simulink model "Sim_Forcing_003h_expe_infra5_full_control4"  (Simulink 7.4)
settings: Solver=FixedStepDiscrete  StartTime=0.0  StopTime=inf  FixedStep=0.004  RelTol=1e-3
undefined symbols (not defined in the file or in its folder): DiscIntNeverNeededParam
libraries: simulink x28, gt_rt_lib x22, xpcutilitieslib x4, xpclib x2, dspswit3 x1
(part 2 of 4)

== system Sim_Forcing_003h_expe_infra5_full_control4/Data to Control Node 12/06/15/Interaction device from VIS (Stick)  ==
  Display2 : Display
  Display4 : Display
  Display5 : Display
  Error : Display
  GT-RT UDP  Read : gt_rt_lib/GT-RT UDP  Controller  uri='gtp://localhost/udp?port=9600'
  GT-RT UDP RX : gt_rt_lib/GT-RT UDP RX  uri='gtp://localhost/udp?port=9600'  receive_buffer_size=28  timeout=0  sample_time=0.004
  Terminator : Terminator
  Unpack : xpclib/UDP/Unpack  dimensions={3,8,1,1}  datatypes={'single','uint8','single','single'}  byteAlign=1
  Stick Out : Outport  OutDataType=fixdt(1, 16)  OutScaling=2^0
  Buttons : Outport  Port=2  OutDataType=fixdt(1, 16)  OutScaling=2^0
  Speed_Test_VIS_Send : Outport  Port=3  OutDataType=fixdt(1, 16)  OutScaling=2^0
  for_delay_calc : Outport  Port=4  OutDataType=fixdt(1, 16)  OutScaling=2^0
  wires:
  GT-RT UDP RX/2 -> Display2/1
  GT-RT UDP RX/6 -> Error/1
  GT-RT UDP RX/5 -> Display4/1
  GT-RT UDP RX/4 -> Display5/1
  GT-RT UDP RX/1 -> Unpack/1
  GT-RT UDP RX/3 -> Terminator/1
  Unpack/1 -> Stick Out/1
  Unpack/2 -> Buttons/1
  Unpack/3 -> Speed_Test_VIS_Send/1
  Unpack/4 -> for_delay_calc/1

== system Sim_Forcing_003h_expe_infra5_full_control4/Handshake CAN/If Action Subsystem ==
  Action Port : ActionPort
  GT-RT CAN TX : gt_rt_lib/GT-RT CAN TX  uri='gt_rt_dev://localhost/dev/can0#0'  mff=MFF_11_DAT
  TX CAN ID1 : Constant  Value=hex2dec('100')  OutDataTypeMode=uint32  OutDataType=sfix(16)  OutScaling=2^0  OutDataTypeStr=uint32
  TX Data : Constant  OutDataTypeMode=uint8  OutDataType=sfix(16)  OutScaling=2^0  OutDataTypeStr=uint8
  wires:
  TX CAN ID1/1 -> GT-RT CAN TX/1
  TX Data/1 -> GT-RT CAN TX/2

== system Sim_Forcing_003h_expe_infra5_full_control4/Handshake CAN/If Action Subsystem1 ==
  Action Port : ActionPort  ActionType=then
  GT-RT CAN TX : gt_rt_lib/GT-RT CAN TX  uri='gt_rt_dev://localhost/dev/can0#0'  mff=MFF_11_DAT
  TX CAN ID1 : Constant  Value=hex2dec('100')  OutDataTypeMode=uint32  OutDataType=sfix(16)  OutScaling=2^0  OutDataTypeStr=uint32
  TX Data : Constant  OutDataTypeMode=uint8  OutDataType=sfix(16)  OutScaling=2^0  OutDataTypeStr=uint8
  wires:
  TX CAN ID1/1 -> GT-RT CAN TX/1
  TX Data/1 -> GT-RT CAN TX/2

== system Sim_Forcing_003h_expe_infra5_full_control4/Joint Controller (May 7, 2015)1/Forward Kinematics ==
  J_ANG_ACT : Inport
  Data Type Conversion4 : DataTypeConversion  OutDataTypeMode=double  OutDataType=fixdt(1, 16)  OutScaling=2^0  OutDataTypeStr=double
  Demux1 : Demux  Outputs=[3,1,1,1]
  Embedded MATLAB Function : Stateflow chart
  KUKA2NED : Subsystem
  Mux : Mux  Inputs=3
  6-DOF_ACT : Outport
  roll_pitch_yaw_act : Outport  Port=2
  wires:
  KUKA2NED/1(NED) -> Embedded MATLAB Function/1(vec)
  Embedded MATLAB Function/1(out) -> 6-DOF_ACT/1, Data Type Conversion4/1
  J_ANG_ACT/1 -> KUKA2NED/1(KUKA)
  Demux1/3 -> Mux/2
  Demux1/2 -> Mux/1
  Mux/1 -> roll_pitch_yaw_act/1
  Data Type Conversion4/1 -> Demux1/1
  Demux1/4 -> Mux/3

== system Sim_Forcing_003h_expe_infra5_full_control4/Joint Controller (May 7, 2015)1/Increments ==
  J_ANG : Inport
  Sum6 : Sum  Inputs=|+-  OutDataType=fixdt(1, 16)  OutScaling=2^0
  Unit Delay6 : UnitDelay  X0=[0 50 -68 0 18 0]'  SampleTime=-1
  J_ANG_INC : Outport
  wires:
  Unit Delay6/1 -> Sum6/2
  J_ANG/1 -> Unit Delay6/1, Sum6/1
  Sum6/1 -> J_ANG_INC/1

== system Sim_Forcing_003h_expe_infra5_full_control4/Joint Controller (May 7, 2015)1/Inverse Kinematics May 6, 2015 ==
  note: Delay of 0.004s to initialize the currect step with the value of J_ANG of the previous loop
  6-DOF : Inport  OutDataType=fixdt(1, 16)  OutScaling=2^0
  Activate_full_inverse : Inport  Port=2  OutDataType=fixdt(1, 16)  OutScaling=2^0
  6_DOF_ACT : Inport  Port=3  OutDataType=fixdt(1, 16)  OutScaling=2^0
  Constant : Constant  OutDataType=fixdt(1, 16)  OutScaling=2^0
  Demux : Demux  Outputs=[6 1]
  Ground : Ground
  Inverse Kinematics : Subsystem
  Mux : Mux  Inputs=2
  NED2KUKA : Subsystem
  Scope1 : Scope
      settings: YMin=-50  YMax=70  SaveName=ScopeData4
  Simplified Inverse Kinematics : Subsystem
  Starting Joint Angles KUKA : Constant  Value=[0 -50 68 0 -18 15.89]'  OutDataType=fixdt(1, 16)  OutScaling=2^0
  Starting Joint Angles NED : Constant  Value=[0 50 -68 0 18 0]'  OutDataType=fixdt(1, 16)  OutScaling=2^0
  Switch : Switch  Criteria=u2 > Threshold  OutDataType=fixdt(1, 16)  OutScaling=2^0
  Switch1 : Switch  Criteria=u2 > Threshold  OutDataType=fixdt(1, 16)  OutScaling=2^0
  Unit Delay : UnitDelay  X0=[0 50 -68 0 18 0]'  SampleTime=-1
  J_ANG : Outport  OutDataType=fixdt(1, 16)  OutScaling=2^0
  N : Outport  Port=2  OutDataType=fixdt(1, 16)  OutScaling=2^0
  wires:
  NED2KUKA/1(KUKA) -> Scope1/1, J_ANG/1
  6-DOF/1 -> Mux/1
  Unit Delay/1 -> Mux/2
  Demux/1 -> NED2KUKA/1(NED), Unit Delay/1
  Demux/2 -> N/1
  Simplified Inverse Kinematics/1(out) -> Switch/1
  Inverse Kinematics/1(out) -> Switch/3
  Switch/1 -> Demux/1
  Mux/1 -> Inverse Kinematics/1(vec), Simplified Inverse Kinematics/2(vec)
  Activate_full_inverse/1 -> Inverse Kinematics/2(Activate full inverse), Switch1/2
  Ground/1 -> Switch1/1
  Switch1/1 -> Simplified Inverse Kinematics/1(activate simplified), Switch/2
  Constant/1 -> Switch1/3
  6_DOF_ACT/1 -> Inverse Kinematics/3(6_DOF_ACT)

== system Sim_Forcing_003h_expe_infra5_full_control4/Joint Controller (May 7, 2015)1/Subtract psi offset ==
  Psi_Offset : Inport
  J_ANG_ACT : Inport  Port=2
  Data Type Conversion : DataTypeConversion  OutDataTypeMode=double  OutDataType=fixdt(1, 16)  OutScaling=2^0  OutDataTypeStr=double
  Demux1 : Demux  Outputs=[1,5]
  Mux1 : Mux  Inputs=[1,5]
  Sum3 : Sum  Inputs=-+|  OutDataType=fixdt(1, 16)  OutScaling=2^0
  out : Outport
  wires:
  Demux1/1 -> Sum3/2
  Sum3/1 -> Mux1/1
  Demux1/2 -> Mux1/2
  J_ANG_ACT/1 -> Data Type Conversion/1
  Mux1/1 -> out/1
  Data Type Conversion/1 -> Demux1/1
  Psi_Offset/1 -> Sum3/1

== system Sim_Forcing_003h_expe_infra5_full_control4/BEC (May 7, 2015)/CAN Receive/Convert 4*uni8 to int ==
  byte0 : Inport
  byte1 : Inport  Port=2
  byte2 : Inport  Port=3
  byte3 : Inport  Port=4
  Add : Sum  Inputs=++++  OutDataTypeMode=int32  OutDataType=fixdt(1, 16)  OutScaling=2^-10  OutDataTypeStr=int32
  Gain2 : Gain  Gain=256  ParameterDataType=fixdt(1, 16)  ParameterScaling=2^0  OutDataType=fixdt(1, 16)  OutScaling=2^0
  Gain3 : Gain  Gain=2^16  ParameterDataType=fixdt(1, 16)  ParameterScaling=2^0  OutDataType=fixdt(1, 16)  OutScaling=2^0
  Gain4 : Gain  Gain=2^24  ParameterDataType=fixdt(1, 16)  ParameterScaling=2^0  OutDataType=fixdt(1, 16)  OutScaling=2^0
  int : Outport
  wires:
  Gain2/1 -> Add/2
  Gain3/1 -> Add/3
  byte0/1 -> Add/1
  Add/1 -> int/1
  byte1/1 -> Gain2/1
  byte2/1 -> Gain3/1
  byte3/1 -> Gain4/1
  Gain4/1 -> Add/4

== system Sim_Forcing_003h_expe_infra5_full_control4/BEC (May 7, 2015)/CAN Receive/Convert 4*uni8 to int1 ==
  byte0 : Inport
  byte1 : Inport  Port=2
  byte2 : Inport  Port=3
  byte3 : Inport  Port=4
  Add : Sum  Inputs=++++  OutDataTypeMode=int32  OutDataType=fixdt(1, 16)  OutScaling=2^-10  OutDataTypeStr=int32
  Gain2 : Gain  Gain=256  ParameterDataType=fixdt(1, 16)  ParameterScaling=2^0  OutDataType=fixdt(1, 16)  OutScaling=2^0
  Gain3 : Gain  Gain=2^16  ParameterDataType=fixdt(1, 16)  ParameterScaling=2^0  OutDataType=fixdt(1, 16)  OutScaling=2^0
  Gain4 : Gain  Gain=2^24  ParameterDataType=fixdt(1, 16)  ParameterScaling=2^0  OutDataType=fixdt(1, 16)  OutScaling=2^0
  int : Outport
  wires:
  Gain4/1 -> Add/4
  byte3/1 -> Gain4/1
  byte2/1 -> Gain3/1
  byte1/1 -> Gain2/1
  Add/1 -> int/1
  byte0/1 -> Add/1
  Gain3/1 -> Add/3
  Gain2/1 -> Add/2

== system Sim_Forcing_003h_expe_infra5_full_control4/BEC (May 7, 2015)/CAN Receive/Convert 4*uni8 to int2 ==
  byte0 : Inport
  byte1 : Inport  Port=2
  byte2 : Inport  Port=3
  byte3 : Inport  Port=4
  Add : Sum  Inputs=++++  OutDataTypeMode=int32  OutDataType=fixdt(1, 16)  OutScaling=2^-10  OutDataTypeStr=int32
  Gain2 : Gain  Gain=256  ParameterDataType=fixdt(1, 16)  ParameterScaling=2^0  OutDataType=fixdt(1, 16)  OutScaling=2^0
  Gain3 : Gain  Gain=2^16  ParameterDataType=fixdt(1, 16)  ParameterScaling=2^0  OutDataType=fixdt(1, 16)  OutScaling=2^0
  Gain4 : Gain  Gain=2^24  ParameterDataType=fixdt(1, 16)  ParameterScaling=2^0  OutDataType=fixdt(1, 16)  OutScaling=2^0
  int : Outport
  wires:
  Gain2/1 -> Add/2
  Gain3/1 -> Add/3
  byte0/1 -> Add/1
  Add/1 -> int/1
  byte1/1 -> Gain2/1
  byte2/1 -> Gain3/1
  byte3/1 -> Gain4/1
  Gain4/1 -> Add/4

== system Sim_Forcing_003h_expe_infra5_full_control4/BEC (May 7, 2015)/CAN Receive/Convert 4*uni8 to int3 ==
  byte0 : Inport
  byte1 : Inport  Port=2
  byte2 : Inport  Port=3
  byte3 : Inport  Port=4
  Add : Sum  Inputs=++++  OutDataTypeMode=int32  OutDataType=fixdt(1, 16)  OutScaling=2^-10  OutDataTypeStr=int32
  Gain2 : Gain  Gain=256  ParameterDataType=fixdt(1, 16)  ParameterScaling=2^0  OutDataType=fixdt(1, 16)  OutScaling=2^0
  Gain3 : Gain  Gain=2^16  ParameterDataType=fixdt(1, 16)  ParameterScaling=2^0  OutDataType=fixdt(1, 16)  OutScaling=2^0
  Gain4 : Gain  Gain=2^24  ParameterDataType=fixdt(1, 16)  ParameterScaling=2^0  OutDataType=fixdt(1, 16)  OutScaling=2^0
  int : Outport
  wires:
  Gain4/1 -> Add/4
  byte3/1 -> Gain4/1
  byte2/1 -> Gain3/1
  byte1/1 -> Gain2/1
  Add/1 -> int/1
  byte0/1 -> Add/1
  Gain3/1 -> Add/3
  Gain2/1 -> Add/2

== system Sim_Forcing_003h_expe_infra5_full_control4/BEC (May 7, 2015)/CAN Receive/Convert 4*uni8 to int4 ==
  byte0 : Inport
  byte1 : Inport  Port=2
  byte2 : Inport  Port=3
  byte3 : Inport  Port=4
  Add : Sum  Inputs=++++  OutDataTypeMode=int32  OutDataType=fixdt(1, 16)  OutScaling=2^-10  OutDataTypeStr=int32
  Gain2 : Gain  Gain=256  ParameterDataType=fixdt(1, 16)  ParameterScaling=2^0  OutDataType=fixdt(1, 16)  OutScaling=2^0
  Gain3 : Gain  Gain=2^16  ParameterDataType=fixdt(1, 16)  ParameterScaling=2^0  OutDataType=fixdt(1, 16)  OutScaling=2^0
  Gain4 : Gain  Gain=2^24  ParameterDataType=fixdt(1, 16)  ParameterScaling=2^0  OutDataType=fixdt(1, 16)  OutScaling=2^0
  int : Outport
  wires:
  Gain2/1 -> Add/2
  Gain3/1 -> Add/3
  byte0/1 -> Add/1
  Add/1 -> int/1
  byte1/1 -> Gain2/1
  byte2/1 -> Gain3/1
  byte3/1 -> Gain4/1
  Gain4/1 -> Add/4

== system Sim_Forcing_003h_expe_infra5_full_control4/BEC (May 7, 2015)/CAN Receive/Convert 4*uni8 to int5 ==
  byte0 : Inport
  byte1 : Inport  Port=2
  byte2 : Inport  Port=3
  byte3 : Inport  Port=4
  Add : Sum  Inputs=++++  OutDataTypeMode=int32  OutDataType=fixdt(1, 16)  OutScaling=2^-10  OutDataTypeStr=int32
  Gain2 : Gain  Gain=256  ParameterDataType=fixdt(1, 16)  ParameterScaling=2^0  OutDataType=fixdt(1, 16)  OutScaling=2^0
  Gain3 : Gain  Gain=2^16  ParameterDataType=fixdt(1, 16)  ParameterScaling=2^0  OutDataType=fixdt(1, 16)  OutScaling=2^0
  Gain4 : Gain  Gain=2^24  ParameterDataType=fixdt(1, 16)  ParameterScaling=2^0  OutDataType=fixdt(1, 16)  OutScaling=2^0
  int : Outport
  wires:
  Gain4/1 -> Add/4
  byte3/1 -> Gain4/1
  byte2/1 -> Gain3/1
  byte1/1 -> Gain2/1
  Add/1 -> int/1
  byte0/1 -> Add/1
  Gain3/1 -> Add/3
  Gain2/1 -> Add/2

== system Sim_Forcing_003h_expe_infra5_full_control4/BEC (May 7, 2015)/CAN Send/If Action Subsystem1 ==
  In1 : Inport  OutDataType=fixdt(1, 16)  OutScaling=2^0
  In2 : Inport  Port=2  OutDataType=fixdt(1, 16)  OutScaling=2^0
  In3 : Inport  Port=3  OutDataType=fixdt(1, 16)  OutScaling=2^0
  In4 : Inport  Port=4  OutDataType=fixdt(1, 16)  OutScaling=2^0
  In5 : Inport  Port=5  OutDataType=fixdt(1, 16)  OutScaling=2^0
  In6 : Inport  Port=6  OutDataType=fixdt(1, 16)  OutScaling=2^0
  Action Port : ActionPort  ActionType=then
  "Convert int to 4*uni8 " : Subsystem
  Convert int to 4*uni8 1 : Subsystem
  Convert int to 4*uni8 2 : Subsystem
  Convert int to 4*uni8 3 : Subsystem
  Convert int to 4*uni8 4 : Subsystem
  Convert int to 4*uni8 5 : Subsystem
  GT-RT CAN TX : gt_rt_lib/GT-RT CAN TX  uri='gt_rt_dev://localhost/dev/can0#0'  mff=MFF_11_DAT
  GT-RT CAN TX1 : gt_rt_lib/GT-RT CAN TX  uri='gt_rt_dev://localhost/dev/can0#0'  mff=MFF_11_DAT
  GT-RT CAN TX2 : gt_rt_lib/GT-RT CAN TX  uri='gt_rt_dev://localhost/dev/can0#0'  mff=MFF_11_DAT
  Mux : Mux  Inputs=2
  Mux1 : Mux  Inputs=2
  Mux2 : Mux  Inputs=2
  TX CAN ID1 : Constant  Value=hex2dec('101')  OutDataTypeMode=uint32  OutDataType=sfix(16)  OutScaling=2^0  OutDataTypeStr=uint32
  TX CAN ID2 : Constant  Value=hex2dec('102')  OutDataTypeMode=uint32  OutDataType=sfix(16)  OutScaling=2^0  OutDataTypeStr=uint32
  TX CAN ID3 : Constant  Value=hex2dec('103')  OutDataTypeMode=uint32  OutDataType=sfix(16)  OutScaling=2^0  OutDataTypeStr=uint32
  wires:
  In1/1 -> "Convert int to 4*uni8 "/1(in)
  In2/1 -> Convert int to 4*uni8 1/1(in)
  In3/1 -> Convert int to 4*uni8 2/1(in)
  In4/1 -> Convert int to 4*uni8 3/1(in)
  In5/1 -> Convert int to 4*uni8 4/1(in)
  In6/1 -> Convert int to 4*uni8 5/1(in)
  Mux2/1 -> GT-RT CAN TX2/2
  Convert int to 4*uni8 5/1(out) -> Mux2/2
  Convert int to 4*uni8 4/1(out) -> Mux2/1
  Mux1/1 -> GT-RT CAN TX1/2
  Convert int to 4*uni8 3/1(out) -> Mux1/2
  Convert int to 4*uni8 2/1(out) -> Mux1/1
  Mux/1 -> GT-RT CAN TX/2
  Convert int to 4*uni8 1/1(out) -> Mux/2
  "Convert int to 4*uni8 "/1(out) -> Mux/1
  TX CAN ID3/1 -> GT-RT CAN TX2/1
  TX CAN ID2/1 -> GT-RT CAN TX1/1
  TX CAN ID1/1 -> GT-RT CAN TX/1

== system Sim_Forcing_003h_expe_infra5_full_control4/BEC (May 7, 2015)/Software limit switches/Subsystem ==
  In1 : Inport
  act : Inport  Port=2
  Abs1 : Abs  OutDataType=fixdt(1, 16)  OutScaling=2^0
  Abs2 : Abs  OutDataType=fixdt(1, 16)  OutScaling=2^0
  Add1 : Sum  Inputs=+-  OutDataType=fixdt(1, 16)  OutScaling=2^-10
  Add2 : Sum  Inputs=-+  OutDataType=fixdt(1, 16)  OutScaling=2^-10
  Display : Display
  Display2 : Display
  If Action Subsystem : Subsystem  TreatAsAtomicUnit=on
  If Action Subsystem1 : Subsystem  TreatAsAtomicUnit=on
  If2 : If
  NSEA1 : Constant  Value=-160  OutDataType=fixdt(1, 16)  OutScaling=2^0
  PSEA1 : Constant  Value=160  OutDataType=fixdt(1, 16)  OutScaling=2^0
  Switch : Switch  Criteria=u2 > Threshold  OutDataType=fixdt(1, 16)  OutScaling=2^0
  Switch1 : Switch  Criteria=u2 ~= 0  OutDataType=fixdt(1, 16)  OutScaling=2^0
  Out1 : Outport
  wires:
  If Action Subsystem1/1(Out1) -> Switch/3
  If Action Subsystem/1(Out1) -> Display/1, Switch/1
  Abs1/1 -> If Action Subsystem1/2(dif)
  If2/2 -> If Action Subsystem1/Action
  If2/1 -> If Action Subsystem/Action
  In1/1 -> If2/1, If Action Subsystem/2(Inc), If Action Subsystem1/1(Inc), Switch/2, Switch1/2, Switch1/3
  Abs2/1 -> If Action Subsystem/1(dif)
  NSEA1/1 -> Add1/2
  PSEA1/1 -> Add2/1
  Add1/1 -> Abs1/1
  Add2/1 -> Abs2/1
  Switch/1 -> Switch1/1
  Switch1/1 -> Out1/1, Display2/1
  act/1 -> Add1/1, Add2/2

== system Sim_Forcing_003h_expe_infra5_full_control4/BEC (May 7, 2015)/Software limit switches/Subsystem1 ==
  In1 : Inport
  act : Inport  Port=2
  Abs1 : Abs  OutDataType=fixdt(1, 16)  OutScaling=2^0
  Abs2 : Abs  OutDataType=fixdt(1, 16)  OutScaling=2^0
  Add1 : Sum  Inputs=+-  OutDataType=fixdt(1, 16)  OutScaling=2^-10
  Add2 : Sum  Inputs=-+  OutDataType=fixdt(1, 16)  OutScaling=2^-10
  If Action Subsystem : Subsystem  TreatAsAtomicUnit=on
  If Action Subsystem1 : Subsystem  TreatAsAtomicUnit=on
  If2 : If
  NSEA1 : Constant  Value=-130  OutDataType=fixdt(1, 16)  OutScaling=2^0
  PSEA1 : Constant  Value=20  OutDataType=fixdt(1, 16)  OutScaling=2^0
  Switch : Switch  OutDataType=fixdt(1, 16)  OutScaling=2^0
  Switch1 : Switch  Criteria=u2 ~= 0  OutDataType=fixdt(1, 16)  OutScaling=2^0
  Out1 : Outport
  wires:
  act/1 -> Add1/1, Add2/2
  Add2/1 -> Abs2/1
  Add1/1 -> Abs1/1
  PSEA1/1 -> Add2/1
  NSEA1/1 -> Add1/2
  Abs2/1 -> If Action Subsystem/1(dif)
  In1/1 -> If Action Subsystem1/1(Inc), If Action Subsystem/2(Inc), Switch/2, Switch1/2, Switch1/3, If2/1
  If2/1 -> If Action Subsystem/Action
  If2/2 -> If Action Subsystem1/Action
  Abs1/1 -> If Action Subsystem1/2(dif)
  If Action Subsystem/1(Out1) -> Switch/1
  If Action Subsystem1/1(Out1) -> Switch/3
  Switch/1 -> Switch1/1
  Switch1/1 -> Out1/1

== system Sim_Forcing_003h_expe_infra5_full_control4/BEC (May 7, 2015)/Software limit switches/Subsystem2 ==
  In1 : Inport
  act : Inport  Port=2
  Abs1 : Abs  OutDataType=fixdt(1, 16)  OutScaling=2^0
  Abs2 : Abs  OutDataType=fixdt(1, 16)  OutScaling=2^0
  Add1 : Sum  Inputs=+-  OutDataType=fixdt(1, 16)  OutScaling=2^-10
  Add2 : Sum  Inputs=-+  OutDataType=fixdt(1, 16)  OutScaling=2^-10
  If Action Subsystem : Subsystem  TreatAsAtomicUnit=on
  If Action Subsystem1 : Subsystem  TreatAsAtomicUnit=on
  If2 : If
  NSEA1 : Constant  Value=-88  OutDataType=fixdt(1, 16)  OutScaling=2^0
  PSEA1 : Constant  Value=88  OutDataType=fixdt(1, 16)  OutScaling=2^0
  Switch : Switch  OutDataType=fixdt(1, 16)  OutScaling=2^0
  Switch1 : Switch  Criteria=u2 ~= 0  OutDataType=fixdt(1, 16)  OutScaling=2^0
  Out1 : Outport
  wires:
  If Action Subsystem1/1(Out1) -> Switch/3
  If Action Subsystem/1(Out1) -> Switch/1
  Abs1/1 -> If Action Subsystem1/2(dif)
  If2/2 -> If Action Subsystem1/Action
  If2/1 -> If Action Subsystem/Action
  In1/1 -> If2/1, If Action Subsystem/2(Inc), If Action Subsystem1/1(Inc), Switch/2, Switch1/2, Switch1/3
  Abs2/1 -> If Action Subsystem/1(dif)
  NSEA1/1 -> Add1/2
  PSEA1/1 -> Add2/1
  Add1/1 -> Abs1/1
  Add2/1 -> Abs2/1
  act/1 -> Add1/1, Add2/2
  Switch/1 -> Switch1/1
  Switch1/1 -> Out1/1

== system Sim_Forcing_003h_expe_infra5_full_control4/BEC (May 7, 2015)/Software limit switches/Subsystem3 ==
  In1 : Inport
  act : Inport  Port=2
  Abs1 : Abs  OutDataType=fixdt(1, 16)  OutScaling=2^0
  Abs2 : Abs  OutDataType=fixdt(1, 16)  OutScaling=2^0
  Add1 : Sum  Inputs=+-  OutDataType=fixdt(1, 16)  OutScaling=2^-10
  Add2 : Sum  Inputs=-+  OutDataType=fixdt(1, 16)  OutScaling=2^-10
  If Action Subsystem : Subsystem  TreatAsAtomicUnit=on
  If Action Subsystem1 : Subsystem  TreatAsAtomicUnit=on
  If2 : If
  NSEA1 : Constant  Value=-350  OutDataType=fixdt(1, 16)  OutScaling=2^0
  PSEA1 : Constant  Value=350  OutDataType=fixdt(1, 16)  OutScaling=2^0
  Switch : Switch  OutDataType=fixdt(1, 16)  OutScaling=2^0
  Switch1 : Switch  Criteria=u2 ~= 0  OutDataType=fixdt(1, 16)  OutScaling=2^0
  Out1 : Outport
  wires:
  Add2/1 -> Abs2/1
  Add1/1 -> Abs1/1
  PSEA1/1 -> Add2/1
  NSEA1/1 -> Add1/2
  Abs2/1 -> If Action Subsystem/1(dif)
  In1/1 -> If Action Subsystem1/1(Inc), If Action Subsystem/2(Inc), Switch/2, Switch1/2, Switch1/3, If2/1
  If2/1 -> If Action Subsystem/Action
  If2/2 -> If Action Subsystem1/Action
  act/1 -> Add2/2, Add1/1
  Abs1/1 -> If Action Subsystem1/2(dif)
  If Action Subsystem/1(Out1) -> Switch/1
  If Action Subsystem1/1(Out1) -> Switch/3
  Switch/1 -> Switch1/1
  Switch1/1 -> Out1/1

== system Sim_Forcing_003h_expe_infra5_full_control4/BEC (May 7, 2015)/Software limit switches/Subsystem4 ==
  In1 : Inport
  act : Inport  Port=2
  Abs1 : Abs  OutDataType=fixdt(1, 16)  OutScaling=2^0
  Abs2 : Abs  OutDataType=fixdt(1, 16)  OutScaling=2^0
  Add1 : Sum  Inputs=+-  OutDataType=fixdt(1, 16)  OutScaling=2^-10
  Add2 : Sum  Inputs=-+  OutDataType=fixdt(1, 16)  OutScaling=2^-10
  If Action Subsystem : Subsystem  TreatAsAtomicUnit=on
  If Action Subsystem1 : Subsystem  TreatAsAtomicUnit=on
  If2 : If
  NSEA1 : Constant  Value=-61  OutDataType=fixdt(1, 16)  OutScaling=2^0
  PSEA1 : Constant  Value=61  OutDataType=fixdt(1, 16)  OutScaling=2^0
  Switch : Switch  OutDataType=fixdt(1, 16)  OutScaling=2^0
  Switch1 : Switch  Criteria=u2 ~= 0  OutDataType=fixdt(1, 16)  OutScaling=2^0
  Out1 : Outport
  wires:
  If Action Subsystem/1(Out1) -> Switch/1
  Abs1/1 -> If Action Subsystem1/2(dif)
  If2/2 -> If Action Subsystem1/Action
  If2/1 -> If Action Subsystem/Action
  In1/1 -> If2/1, If Action Subsystem/2(Inc), If Action Subsystem1/1(Inc), Switch/2, Switch1/2, Switch1/3
  Abs2/1 -> If Action Subsystem/1(dif)
  NSEA1/1 -> Add1/2
  PSEA1/1 -> Add2/1
  Add1/1 -> Abs1/1
  Add2/1 -> Abs2/1
  If Action Subsystem1/1(Out1) -> Switch/3
  Switch/1 -> Switch1/1
  Switch1/1 -> Out1/1
  act/1 -> Add2/2, Add1/1

== system Sim_Forcing_003h_expe_infra5_full_control4/BEC (May 7, 2015)/Software limit switches/Subsystem5 ==
  In1 : Inport
  act : Inport  Port=2
  Abs1 : Abs  OutDataType=fixdt(1, 16)  OutScaling=2^0
  Abs2 : Abs  OutDataType=fixdt(1, 16)  OutScaling=2^0
  Add1 : Sum  Inputs=+-  OutDataType=fixdt(1, 16)  OutScaling=2^-10
  Add2 : Sum  Inputs=-+  OutDataType=fixdt(1, 16)  OutScaling=2^-10
  If Action Subsystem : Subsystem  TreatAsAtomicUnit=on
  If Action Subsystem1 : Subsystem  TreatAsAtomicUnit=on
  If2 : If
  NSEA1 : Constant  Value=-350  OutDataType=fixdt(1, 16)  OutScaling=2^0
  PSEA1 : Constant  Value=350  OutDataType=fixdt(1, 16)  OutScaling=2^0
  Switch : Switch  OutDataType=fixdt(1, 16)  OutScaling=2^0
  Switch1 : Switch  Criteria=u2 ~= 0  OutDataType=fixdt(1, 16)  OutScaling=2^0
  Out1 : Outport
  wires:
  Add2/1 -> Abs2/1
  Add1/1 -> Abs1/1
  PSEA1/1 -> Add2/1
  NSEA1/1 -> Add1/2
  Abs2/1 -> If Action Subsystem/1(dif)
  In1/1 -> If Action Subsystem1/1(Inc), If Action Subsystem/2(Inc), Switch/2, Switch1/2, Switch1/3, If2/1
  If2/1 -> If Action Subsystem/Action
  If2/2 -> If Action Subsystem1/Action
  Abs1/1 -> If Action Subsystem1/2(dif)
  If Action Subsystem/1(Out1) -> Switch/1
  If Action Subsystem1/1(Out1) -> Switch/3
  Switch/1 -> Switch1/1
  Switch1/1 -> Out1/1
  act/1 -> Add2/2, Add1/1

== system Sim_Forcing_003h_expe_infra5_full_control4/Breaking_Control 20/07/15/Move UP1/Smooth Displacement Second-Order Filter, zeta 0.8 ==
  Step IN Reset on  either : Inport
  T : Inport  Port=2  OutDataType=fixdt(1, 16)  OutScaling=2^0
  (zeta*T_transfer)/pi : Gain  Gain=0.8/pi  ParameterDataType=fixdt(1, 16)  ParameterScaling=2^0  OutDataType=fixdt(1, 16)  OutScaling=2^0
  4*zeta*pi : Gain  Gain=3.2*pi  ParameterDataType=fixdt(1, 16)  ParameterScaling=2^0  OutDataType=fixdt(1, 16)  OutScaling=2^0
  4*zeta*pi/T_transfer /s : DiscreteIntegrator  gainval=1  ExternalReset=either  InitialConditionSource=external  SampleTime=0.004  OutDataType=fixdt(1, 16)  OutScaling=2^0  ICPrevOutput=DiscIntNeverNeededParam  ICPrevScaledInput=DiscIntNeverNeededParam
  Discrete Derivative : simulink/Discrete/Discrete Derivative  SystemSampleTime=-1  gainval=1.0  ICPrevScaledInput=0.0  OutMin=[]  OutMax=[]  OutDataType=fixdt(1, 16)  OutScaling=2^-10  DoSatur=off
  Divide : Product  Inputs=*/  OutDataType=fixdt(1, 16)  OutScaling=2^-10
  Divide1 : Product  Inputs=*/  OutDataType=fixdt(1, 16)  OutScaling=2^-10
  For saving position  and velocity until after switchover : UnitDelay  SampleTime=-1
  Product : Product  OutDataType=fixdt(1, 16)  OutScaling=2^0  RndMeth=Zero
  Sum1 : Sum  Inputs=|+-  OutDataType=fixdt(1, 16)  OutScaling=2^0
  Sum2 : Sum  Inputs=-+|  OutDataType=fixdt(1, 16)  OutScaling=2^0
  pi/(zeta*T_transfer)/s : DiscreteIntegrator  gainval=1  ExternalReset=either  InitialConditionSource=external  SampleTime=0.004  OutDataType=fixdt(1, 16)  OutScaling=2^0  ICPrevOutput=DiscIntNeverNeededParam  ICPrevScaledInput=DiscIntNeverNeededParam
  pi/zeta : Gain  Gain=pi/0.8  ParameterDataType=fixdt(1, 16)  ParameterScaling=2^0  OutDataType=fixdt(1, 16)  OutScaling=2^0
  Out : Outport
  wires:
  Discrete Derivative/1 -> Product/2
  Product/1 -> (zeta*T_transfer)/pi/1
  Divide/1 -> 4*zeta*pi/1
  Divide1/1 -> pi/zeta/1
  pi/zeta/1 -> pi/(zeta*T_transfer)/s/1
  pi/(zeta*T_transfer)/s/1 -> Sum2/1, Out/1, For saving position  and velocity until after switchover/1
  4*zeta*pi/T_transfer /s/1 -> Divide1/1, Sum1/2
  Sum1/1 -> Divide/1
  4*zeta*pi/1 -> 4*zeta*pi/T_transfer /s/1
  T/1 -> [T]
  Step IN Reset on  either/1 -> [Step], Sum2/2
  [Step] -> 4*zeta*pi/T_transfer /s/2
  [Step] -> pi/(zeta*T_transfer)/s/2
  [T] -> Divide/2
  For saving position  and velocity until after switchover/1 -> Discrete Derivative/1, pi/(zeta*T_transfer)/s/3
  [T] -> Product/1
  (zeta*T_transfer)/pi/1 -> 4*zeta*pi/T_transfer /s/3
  [T] -> Divide1/2
  Sum2/1 -> Sum1/1

== system Sim_Forcing_003h_expe_infra5_full_control4/Breaking_Control 20/07/15/Move UP1/add x_offset ==
  x_offset : Inport
  set_in : Inport  Port=2
  Embedded MATLAB Function : Stateflow chart
  set_out : Outport
  wires:
  x_offset/1 -> Embedded MATLAB Function/1(dx)
  Embedded MATLAB Function/1(set_out) -> set_out/1
  set_in/1 -> Embedded MATLAB Function/2(set_in)

== system Sim_Forcing_003h_expe_infra5_full_control4/Breaking_Control 20/07/15/Move_cabin/Subsystem ==
  com_or : Inport
  start_zeroing : Inport  Port=2
  connect_x : Inport  Port=3
  connect_z : Inport  Port=4
  Display4 : Display
  Display5 : Display
  Embedded MATLAB Function3 : Stateflow chart
  Fcn : Fcn  Expr=abs(u(1))+abs(u(2))+abs(u(3))+abs(u(4))
  Logical Operator : Logic  AllPortsSameDT=off  OutDataTypeMode=boolean  LogicDataType=fixdt(0, 8)  OutDataTypeStr=boolean
  Logical Operator1 : Logic  Operator=OR  AllPortsSameDT=off  OutDataTypeMode=boolean  LogicDataType=fixdt(0, 8)  OutDataTypeStr=boolean
  Logical Operator2 : Logic  Operator=NOT  AllPortsSameDT=off  OutDataTypeMode=boolean  LogicDataType=fixdt(0, 8)  OutDataTypeStr=boolean
  Logical Operator3 : Logic  AllPortsSameDT=off  OutDataTypeMode=boolean  LogicDataType=fixdt(0, 8)  OutDataTypeStr=boolean
  Logical Operator4 : Logic  AllPortsSameDT=off  OutDataTypeMode=boolean  LogicDataType=fixdt(0, 8)  OutDataTypeStr=boolean
  Logical Operator5 : Logic  Operator=OR  AllPortsSameDT=off  OutDataTypeMode=boolean  LogicDataType=fixdt(0, 8)  OutDataTypeStr=boolean
  Logical Operator6 : Logic  Operator=NOT  AllPortsSameDT=off  OutDataTypeMode=boolean  LogicDataType=fixdt(0, 8)  OutDataTypeStr=boolean
  Relational Operator : RelationalOperator  Operator=<=  LogicOutDataTypeMode=boolean  LogicDataType=fixdt(0, 8)  OutDataTypeStr=boolean
  gain : Constant  Value=0.004
  flag_reset : Outport  OutDataType=fixdt(1, 16)  OutScaling=2^0
  wires:
  gain/1 -> Relational Operator/2
  Logical Operator/1 -> Display4/1, flag_reset/1
  com_or/1 -> Embedded MATLAB Function3/1(com_or), Fcn/1
  Embedded MATLAB Function3/1(max_tilt) -> Relational Operator/1
  start_zeroing/1 -> Logical Operator3/1, Logical Operator5/1
  connect_x/1 -> Logical Operator6/1, Logical Operator3/2
  connect_z/1 -> Logical Operator2/1
  Logical Operator2/1 -> Logical Operator1/2
  Logical Operator3/1 -> Logical Operator1/1
  Logical Operator1/1 -> Logical Operator/2
  Relational Operator/1 -> Logical Operator4/1
  Logical Operator4/1 -> Logical Operator/1
  Logical Operator5/1 -> Logical Operator4/2
  Logical Operator6/1 -> Logical Operator5/2

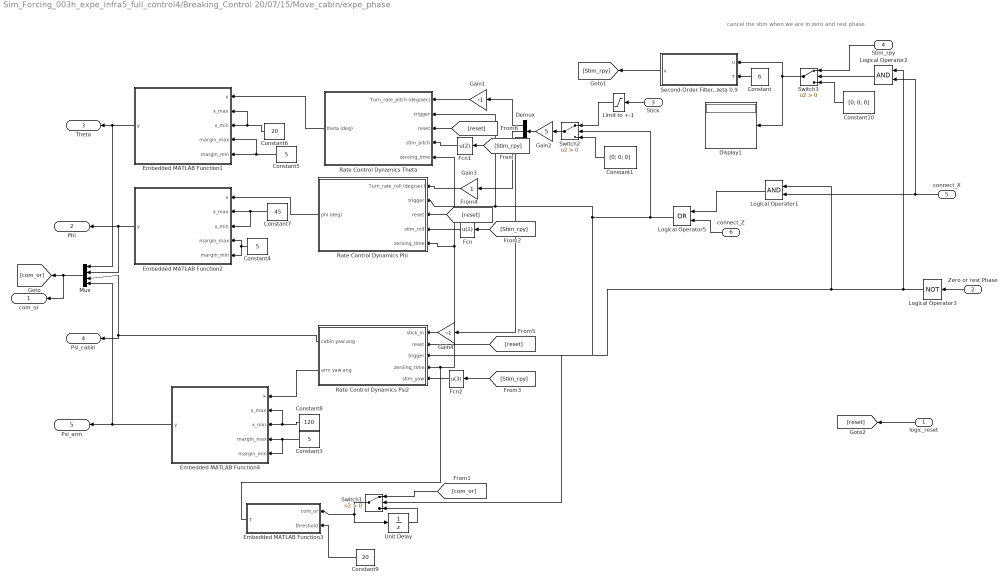
== system Sim_Forcing_003h_expe_infra5_full_control4/Breaking_Control 20/07/15/Move_cabin/expe_phase ==
  note: cancel the stim when we are in zero and rest phase
  logic_reset : Inport
  Zero or rest Phase : Inport  Port=2  OutDataType=fixdt(1, 16)  OutScaling=2^0
  Stick : Inport  Port=3
  Stim_rpy : Inport  Port=4
  connect_X : Inport  Port=5  OutDataType=fixdt(1, 16)  OutScaling=2^0
  connect_Z : Inport  Port=6  OutDataType=fixdt(1, 16)  OutScaling=2^0
  Constant : Constant  Value=6  OutDataType=fixdt(1, 16)  OutScaling=2^0
  Constant1 : Constant  Value=[0; 0; 0]  OutDataType=fixdt(1, 16)  OutScaling=2^0
  Constant10 : Constant  Value=[0; 0; 0]  OutDataType=fixdt(1, 16)  OutScaling=2^0
  Constant3 : Constant  Value=5  OutDataType=fixdt(1, 16)  OutScaling=2^0
  Constant4 : Constant  Value=5  OutDataType=fixdt(1, 16)  OutScaling=2^0
  Constant5 : Constant  Value=5  OutDataType=fixdt(1, 16)  OutScaling=2^0
  Constant6 : Constant  Value=20  OutDataType=fixdt(1, 16)  OutScaling=2^0
  Constant7 : Constant  Value=45  OutDataType=fixdt(1, 16)  OutScaling=2^0
  Constant8 : Constant  Value=120  OutDataType=fixdt(1, 16)  OutScaling=2^0
  Constant9 : Constant  Value=20  OutDataType=fixdt(1, 16)  OutScaling=2^0
  Demux : Demux  Outputs=3
  Display1 : Display
  Embedded MATLAB Function1 : Stateflow chart
  Embedded MATLAB Function2 : Stateflow chart
  Embedded MATLAB Function3 : Stateflow chart
  Embedded MATLAB Function4 : Stateflow chart
  Fcn : Fcn  Expr=u(1)
  Fcn1 : Fcn  Expr=u(2)
  Fcn2 : Fcn  Expr=u(3)
  Gain1 : Gain  Gain=-1  ParameterDataType=fixdt(1, 16)  ParameterScaling=2^0  OutDataType=fixdt(1, 16)  OutScaling=2^0
  Gain2 : Gain  Gain=5  ParameterDataType=fixdt(1, 16)  ParameterScaling=2^0  OutDataType=fixdt(1, 16)  OutScaling=2^0
  Gain3 : Gain  ParameterDataType=fixdt(1, 16)  ParameterScaling=2^0  OutDataType=fixdt(1, 16)  OutScaling=2^0
  Gain4 : Gain  Gain=-1  ParameterDataType=fixdt(1, 16)  ParameterScaling=2^0  OutDataType=fixdt(1, 16)  OutScaling=2^0
  Limit to +-1 : Saturate  UpperLimit=1  LowerLimit=-1  OutDataType=fixdt(1, 16)  OutScaling=2^0
  Logical Operator1 : Logic  AllPortsSameDT=off  OutDataTypeMode=boolean  LogicDataType=fixdt(0, 8)  OutDataTypeStr=boolean
  Logical Operator2 : Logic  AllPortsSameDT=off  OutDataTypeMode=boolean  LogicDataType=fixdt(0, 8)  OutDataTypeStr=boolean
  Logical Operator3 : Logic  Operator=NOT  AllPortsSameDT=off  OutDataTypeMode=boolean  LogicDataType=fixdt(0, 8)  OutDataTypeStr=boolean
  Logical Operator5 : Logic  Operator=OR  AllPortsSameDT=off  OutDataTypeMode=boolean  LogicDataType=fixdt(0, 8)  OutDataTypeStr=boolean
  Mux : Mux
  Rate Control Dynamics Phi : Subsystem
  Rate Control Dynamics Psi2 : Subsystem
  Rate Control Dynamics Theta : Subsystem
  "Second-Order Filter, zeta 0.9" : Subsystem
  Switch1 : Switch  Criteria=u2 > Threshold  OutDataType=fixdt(1, 16)  OutScaling=2^0
  Switch2 : Switch  Criteria=u2 > Threshold  OutDataType=fixdt(1, 16)  OutScaling=2^0
  Switch3 : Switch  Criteria=u2 > Threshold  OutDataType=fixdt(1, 16)  OutScaling=2^0
  Unit Delay : UnitDelay  X0=[0 0 0 0]  SampleTime=-1
  com_or : Outport
  Phi : Outport  Port=2
  Theta : Outport  Port=3
  Psi_cabin : Outport  Port=4
  Psi_arm : Outport  Port=5
  wires:
  Gain2/1 -> Demux/1
  Demux/1 -> Gain1/1
  Demux/2 -> Gain3/1
  Switch2/1 -> Gain2/1
  Stick/1 -> Limit to +-1/1
  Demux/3 -> Gain4/1
  Zero or rest Phase/1 -> Logical Operator3/1
  Rate Control Dynamics Psi2/1(cabin yaw ang) -> Psi_cabin/1, Mux/3
  Embedded MATLAB Function1/1(y) -> Theta/1, Mux/1
  Constant7/1 -> Embedded MATLAB Function2/2(x_max), Embedded MATLAB Function2/3(x_min)
  Rate Control Dynamics Phi/1(phi (deg)) -> Embedded MATLAB Function2/1(x)
  Embedded MATLAB Function2/1(y) -> Phi/1, Mux/2
  Constant3/1 -> Embedded MATLAB Function4/4(margin_max), Embedded MATLAB Function4/5(margin_min)
  Constant8/1 -> Embedded MATLAB Function4/3(x_min), Embedded MATLAB Function4/2(x_max)
  Embedded MATLAB Function4/1(y) -> Psi_arm/1, Mux/4
  Constant4/1 -> Embedded MATLAB Function2/4(margin_max), Embedded MATLAB Function2/5(margin_min)
  Constant5/1 -> Embedded MATLAB Function1/4(margin_max), Embedded MATLAB Function1/5(margin_min)
  Constant6/1 -> Embedded MATLAB Function1/3(x_min), Embedded MATLAB Function1/2(x_max)
  Rate Control Dynamics Theta/1(theta (deg)) -> Embedded MATLAB Function1/1(x)
  Rate Control Dynamics Psi2/2(arm yaw ang) -> Embedded MATLAB Function4/1(x)
  Constant9/1 -> Embedded MATLAB Function3/2(threshold)
  Switch1/1 -> Embedded MATLAB Function3/1(com_or), Unit Delay/1
  Unit Delay/1 -> Switch1/3
  Embedded MATLAB Function3/1(T) -> Rate Control Dynamics Psi2/4(zeroing_time), Rate Control Dynamics Phi/5(zeroing_time), Rate Control Dynamics Theta/5(zeroing_time)
  Mux/1 -> [com_or], com_or/1
  [com_or] -> Switch1/1
  Gain3/1 -> Rate Control Dynamics Phi/1(Turn_rate_roll (deg/sec))
  Gain4/1 -> Rate Control Dynamics Psi2/1(stick_in)
  [Stim_rpy] -> Fcn/1
  [Stim_rpy] -> Fcn1/1
  Fcn2/1 -> Rate Control Dynamics Psi2/5(stim_yaw)
  [Stim_rpy] -> Fcn2/1
  Logical Operator3/1 -> Logical Operator2/1, Logical Operator1/1, Switch1/2
  Logical Operator1/1 -> Logical Operator5/1
  Constant1/1 -> Switch2/3
  Limit to +-1/1 -> Switch2/1
  connect_X/1 -> Logical Operator1/2, Logical Operator2/2
  Constant10/1 -> Switch3/3
  Logical Operator2/1 -> Switch3/2
  Switch3/1 -> Display1/1, "Second-Order Filter, zeta 0.9"/1(u)
  Stim_rpy/1 -> Switch3/1
  logic_reset/1 -> [reset]
  [reset] -> Rate Control Dynamics Phi/3(reset)
  [reset] -> Rate Control Dynamics Psi2/2("reset ")
  [reset] -> Rate Control Dynamics Theta/3(reset)
  Gain1/1 -> Rate Control Dynamics Theta/1(Turn_rate_pitch (deg/sec))
  Fcn1/1 -> Rate Control Dynamics Theta/4(stim_pitch)
  Fcn/1 -> Rate Control Dynamics Phi/4(stim_roll)
  Logical Operator5/1 -> Rate Control Dynamics Phi/2(trigger), Rate Control Dynamics Theta/2(trigger), Rate Control Dynamics Psi2/3(trigger), Switch2/2
  connect_Z/1 -> Logical Operator5/2
  Constant/1 -> "Second-Order Filter, zeta 0.9"/2(T)
  "Second-Order Filter, zeta 0.9"/1(x) -> [Stim_rpy]

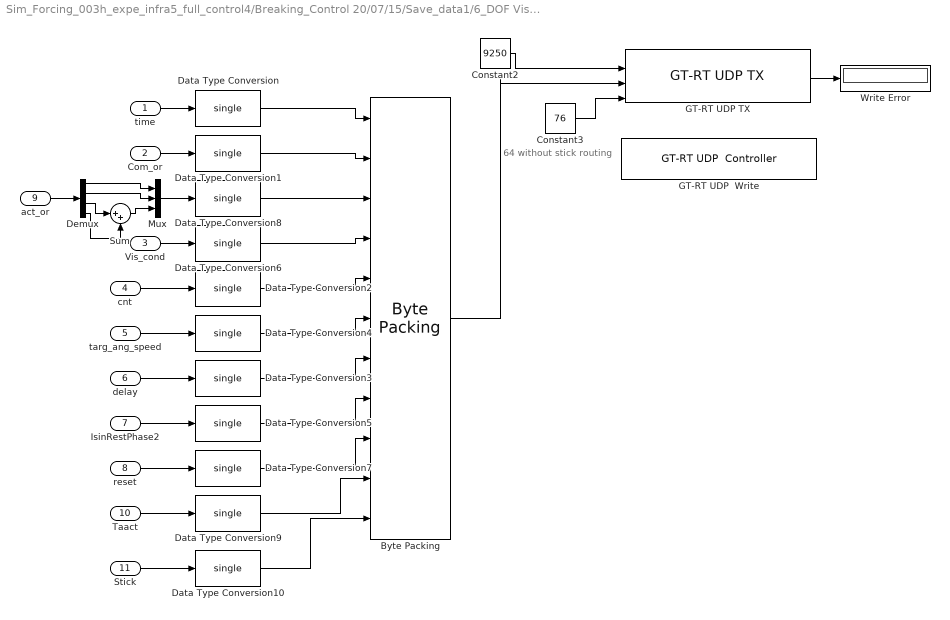
== system Sim_Forcing_003h_expe_infra5_full_control4/Breaking_Control 20/07/15/Save_data1/6_DOF Visual Cab 12/06/15 ==
  note: 64 without stick routing
  time : Inport
  Com_or : Inport  Port=2
  Vis_cond : Inport  Port=3
  cnt : Inport  Port=4
  targ_ang_speed : Inport  Port=5
  delay : Inport  Port=6
  IsinRestPhase2 : Inport  Port=7
  reset : Inport  Port=8
  act_or : Inport  Port=9
  Taact : Inport  Port=10
  Stick : Inport  Port=11
  "Byte Packing " : xpcutilitieslib/Byte Packing   MaskPackedDataType=uint8  MaskUnpackedDataTypes={'single','single','single','single','single','single','single','single','single','single','single'}  MaskAlignment=1
  Constant2 : Constant  Value=9250  OutDataTypeMode=uint16  OutDataType=fixdt(1, 16)  OutScaling=2^0  OutDataTypeStr=uint16
  Constant3 : Constant  Value=76  OutDataTypeMode=uint32  OutDataType=fixdt(1, 16)  OutScaling=2^0  OutDataTypeStr=uint32
  Data Type Conversion{,1..10} (11 alike) : DataTypeConversion  OutDataTypeMode=single  OutDataType=fixdt(1, 16)  OutScaling=2^0  OutDataTypeStr=single
  Demux : Demux
  GT-RT UDP  Write : gt_rt_lib/GT-RT UDP  Controller  uri='gtp://localhost/udp?port=9250'
  GT-RT UDP TX : gt_rt_lib/GT-RT UDP TX  uri='gtp://localhost/udp?port=9250'  hostname='192.168.102.50'
  Mux : Mux  Inputs=3
  Sum : Sum  Inputs=|++  OutDataType=fixdt(1, 16)  OutScaling=2^0
  Write Error : Display
  wires:
  Constant2/1 -> GT-RT UDP TX/2
  GT-RT UDP TX/1 -> Write Error/1
  Constant3/1 -> GT-RT UDP TX/4
  "Byte Packing "/1 -> GT-RT UDP TX/3
  Com_or/1 -> Data Type Conversion1/1
  time/1 -> Data Type Conversion/1
  Data Type Conversion1/1 -> "Byte Packing "/2
  cnt/1 -> Data Type Conversion2/1
  Data Type Conversion/1 -> "Byte Packing "/1
  targ_ang_speed/1 -> Data Type Conversion4/1
  Vis_cond/1 -> Data Type Conversion6/1
  delay/1 -> Data Type Conversion3/1
  IsinRestPhase2/1 -> Data Type Conversion5/1
  reset/1 -> Data Type Conversion7/1
  Data Type Conversion5/1 -> "Byte Packing "/8
  Data Type Conversion7/1 -> "Byte Packing "/9
  Data Type Conversion3/1 -> "Byte Packing "/7
  Data Type Conversion4/1 -> "Byte Packing "/6
  Data Type Conversion2/1 -> "Byte Packing "/5
  Data Type Conversion6/1 -> "Byte Packing "/4
  Data Type Conversion8/1 -> "Byte Packing "/3
  Taact/1 -> Data Type Conversion9/1
  Data Type Conversion9/1 -> "Byte Packing "/10
  Stick/1 -> Data Type Conversion10/1
  Data Type Conversion10/1 -> "Byte Packing "/11
  act_or/1 -> Demux/1
  Demux/1 -> Mux/1
  Demux/2 -> Mux/2
  Mux/1 -> Data Type Conversion8/1
  Demux/3 -> Sum/1
  Demux/4 -> Sum/2
  Sum/1 -> Mux/3

== system Sim_Forcing_003h_expe_infra5_full_control4/Joint Controller (May 7, 2015)1/Forward Kinematics/KUKA2NED ==
  KUKA : Inport
  Constant : Constant  Value=[0 0 0 0 0 15.89]  OutDataType=fixdt(1, 16)  OutScaling=2^0
  Gain : Gain  Gain=[1 -1 -1 -1 -1 -1]  ParameterDataType=fixdt(1, 16)  ParameterScaling=2^0  OutDataType=fixdt(1, 16)  OutScaling=2^0
  Sum : Sum  Inputs=|++  OutDataType=fixdt(1, 16)  OutScaling=2^0
  NED : Outport
  wires:
  Gain/1 -> Sum/1
  KUKA/1 -> Gain/1
  Sum/1 -> NED/1
  Constant/1 -> Sum/2

== system Sim_Forcing_003h_expe_infra5_full_control4/Joint Controller (May 7, 2015)1/Inverse Kinematics May 6, 2015/Inverse Kinematics ==
  note: (6_DOF_ACT - 6_DOF_COM) exp(-0.1t) + 6_DOF_COM
  vec : Inport
  Activate full inverse : Inport  Port=2
  6_DOF_ACT : Inport  Port=3  OutDataType=fixdt(1, 16)  OutScaling=2^0
  Demux : Demux  Outputs=[6,6]
  Discrete-Time Integrator : DiscreteIntegrator  gainval=1  ExternalReset=either  InitialConditionSource=external  SampleTime=-1  OutDataType=fixdt(1, 16)  OutScaling=2^0  ICPrevOutput=DiscIntNeverNeededParam  ICPrevScaledInput=DiscIntNeverNeededParam
  Gain : Gain  Gain=-0.1  ParameterDataType=fixdt(1, 16)  ParameterScaling=2^0  OutDataType=fixdt(1, 16)  OutScaling=2^0
  Mux : Mux  Inputs=2
  Select -6_DOF_COM : Selector  InputPortWidth=12  IndexOptions=Index vector (dialog)  Indices=[1 2 3 4 5 6]  OutputSizes=1
  Sum : Sum  Inputs=|-+  OutDataType=fixdt(1, 16)  OutScaling=2^0
  Sum1 : Sum  Inputs=|++  OutDataType=fixdt(1, 16)  OutScaling=2^0
  full inverse kin : Subsystem
  out : Outport  OutDataType=fixdt(1, 16)  OutScaling=2^0
  wires:
  vec/1 -> Select -6_DOF_COM/1, Demux/1
  full inverse kin/1(out) -> out/1
  Activate full inverse/1 -> full inverse kin/Enable, Discrete-Time Integrator/2
  Discrete-Time Integrator/1 -> Gain/1, Sum1/2
  Gain/1 -> Discrete-Time Integrator/1
  6_DOF_ACT/1 -> Sum/2
  Select -6_DOF_COM/1 -> Sum/1
  Sum/1 -> Discrete-Time Integrator/3
  Demux/2 -> Mux/2
  Demux/1 -> Sum1/1
  Sum1/1 -> Mux/1
  Mux/1 -> full inverse kin/1(vec)

== system Sim_Forcing_003h_expe_infra5_full_control4/Joint Controller (May 7, 2015)1/Inverse Kinematics May 6, 2015/NED2KUKA ==
  NED : Inport
  Constant : Constant  Value=[0 0 0 0 0 15.89]  OutDataType=fixdt(1, 16)  OutScaling=2^0
  Gain : Gain  Gain=[1 -1 -1 -1 -1 -1]  ParameterDataType=fixdt(1, 16)  ParameterScaling=2^0  OutDataType=fixdt(1, 16)  OutScaling=2^0
  Sum : Sum  Inputs=|++  OutDataType=fixdt(1, 16)  OutScaling=2^0
  KUKA : Outport
  wires:
  Gain/1 -> Sum/1
  NED/1 -> Gain/1
  Sum/1 -> KUKA/1
  Constant/1 -> Sum/2

== system Sim_Forcing_003h_expe_infra5_full_control4/Joint Controller (May 7, 2015)1/Inverse Kinematics May 6, 2015/Simplified Inverse Kinematics ==
  note: (A1-A6_ACT - A1-A6_COM) exp(-0.1t) + A1-A6_COM
  note: Selects and sets
      |  A1, A4,A6 to zero
  note: This version has been tested on May 6, 2015
  activate simplified : Inport  OutDataType=fixdt(1, 16)  OutScaling=2^0
  vec : Inport  Port=2  OutDataType=fixdt(1, 16)  OutScaling=2^0
  A1-A6 ACT : Selector  InputPortWidth=12  IndexOptions=Index vector (dialog)  Indices=[7 8 9 10 11 12]  OutputSizes=1
  A1-A6 COM : Subsystem
  Discrete-Time Integrator1 : DiscreteIntegrator  gainval=1  ExternalReset=either  InitialConditionSource=external  SampleTime=-1  OutDataType=fixdt(1, 16)  OutScaling=2^0  ICPrevOutput=DiscIntNeverNeededParam  ICPrevScaledInput=DiscIntNeverNeededParam
  Gain1 : Gain  Gain=-0.1  ParameterDataType=fixdt(1, 16)  ParameterScaling=2^0  OutDataType=fixdt(1, 16)  OutScaling=2^0
  Mux : Mux  Inputs=2
  N : Selector  InputPortWidth=7  IndexOptions=Index vector (dialog)  Indices=7  OutputSizes=1
  Simplified Inverse Kin : Subsystem
  Sum : Sum  Inputs=-+|  OutDataType=fixdt(1, 16)  OutScaling=2^0
  Sum1 : Sum  Inputs=++|  OutDataType=fixdt(1, 16)  OutScaling=2^0
  out : Outport  OutDataType=fixdt(1, 16)  OutScaling=2^0
  wires:
  vec/1 -> Simplified Inverse Kin/1(Vec), A1-A6 ACT/1
  activate simplified/1 -> Simplified Inverse Kin/Enable, Discrete-Time Integrator1/2
  Discrete-Time Integrator1/1 -> Gain1/1, Sum1/2
  Gain1/1 -> Discrete-Time Integrator1/1
  Sum1/1 -> Mux/1
  Sum/1 -> Discrete-Time Integrator1/3
  Mux/1 -> out/1
  A1-A6 ACT/1 -> Sum/2
  Simplified Inverse Kin/1(Out) -> A1-A6 COM/1(vec), N/1
  A1-A6 COM/1(A1-A6 COM) -> Sum/1, Sum1/1
  N/1 -> Mux/2

== system Sim_Forcing_003h_expe_infra5_full_control4/BEC (May 7, 2015)/CAN Send/If Action Subsystem1/Convert int to 4*uni8  ==
  in : Inport
  Gain{1..4} (4 alike) : Gain  ParameterDataType=fixdt(1, 16)  ParameterScaling=2^0  OutDataTypeMode=uint8  OutDataType=fixdt(1, 16)  OutScaling=2^0  OutDataTypeStr=uint8
  Mux : Mux
  Shift Arithmetic : simulink/Logic and Bit Operations/Shift Arithmetic  SystemSampleTime=-1  nBitShiftRight=8  nBinPtShiftRight=0
  Shift Arithmetic1 : simulink/Logic and Bit Operations/Shift Arithmetic  SystemSampleTime=-1  nBitShiftRight=16  nBinPtShiftRight=0
  Shift Arithmetic2 : simulink/Logic and Bit Operations/Shift Arithmetic  SystemSampleTime=-1  nBitShiftRight=24  nBinPtShiftRight=0
  out : Outport
  wires:
  in/1 -> Shift Arithmetic1/1, Gain1/1, Shift Arithmetic/1, Shift Arithmetic2/1
  Shift Arithmetic/1 -> Gain2/1
  Shift Arithmetic1/1 -> Gain3/1
  Shift Arithmetic2/1 -> Gain4/1
  Gain1/1 -> Mux/1
  Gain2/1 -> Mux/2
  Gain3/1 -> Mux/3
  Gain4/1 -> Mux/4
  Mux/1 -> out/1

== system Sim_Forcing_003h_expe_infra5_full_control4/BEC (May 7, 2015)/CAN Send/If Action Subsystem1/Convert int to 4*uni8 1 ==
  in : Inport
  Gain{1..4} (4 alike) : Gain  ParameterDataType=fixdt(1, 16)  ParameterScaling=2^0  OutDataTypeMode=uint8  OutDataType=fixdt(1, 16)  OutScaling=2^0  OutDataTypeStr=uint8
  Mux : Mux
  Shift Arithmetic : simulink/Logic and Bit Operations/Shift Arithmetic  SystemSampleTime=-1  nBitShiftRight=8  nBinPtShiftRight=0
  Shift Arithmetic1 : simulink/Logic and Bit Operations/Shift Arithmetic  SystemSampleTime=-1  nBitShiftRight=16  nBinPtShiftRight=0
  Shift Arithmetic2 : simulink/Logic and Bit Operations/Shift Arithmetic  SystemSampleTime=-1  nBitShiftRight=24  nBinPtShiftRight=0
  out : Outport
  wires:
  Mux/1 -> out/1
  Gain4/1 -> Mux/4
  Gain3/1 -> Mux/3
  Gain2/1 -> Mux/2
  Gain1/1 -> Mux/1
  Shift Arithmetic2/1 -> Gain4/1
  Shift Arithmetic1/1 -> Gain3/1
  Shift Arithmetic/1 -> Gain2/1
  in/1 -> Shift Arithmetic2/1, Shift Arithmetic/1, Gain1/1, Shift Arithmetic1/1

== system Sim_Forcing_003h_expe_infra5_full_control4/BEC (May 7, 2015)/CAN Send/If Action Subsystem1/Convert int to 4*uni8 2 ==
  in : Inport
  Gain{1..4} (4 alike) : Gain  ParameterDataType=fixdt(1, 16)  ParameterScaling=2^0  OutDataTypeMode=uint8  OutDataType=fixdt(1, 16)  OutScaling=2^0  OutDataTypeStr=uint8
  Mux : Mux
  Shift Arithmetic : simulink/Logic and Bit Operations/Shift Arithmetic  SystemSampleTime=-1  nBitShiftRight=8  nBinPtShiftRight=0
  Shift Arithmetic1 : simulink/Logic and Bit Operations/Shift Arithmetic  SystemSampleTime=-1  nBitShiftRight=16  nBinPtShiftRight=0
  Shift Arithmetic2 : simulink/Logic and Bit Operations/Shift Arithmetic  SystemSampleTime=-1  nBitShiftRight=24  nBinPtShiftRight=0
  out : Outport
  wires:
  Mux/1 -> out/1
  Gain4/1 -> Mux/4
  Gain3/1 -> Mux/3
  Gain2/1 -> Mux/2
  Gain1/1 -> Mux/1
  Shift Arithmetic2/1 -> Gain4/1
  Shift Arithmetic1/1 -> Gain3/1
  Shift Arithmetic/1 -> Gain2/1
  in/1 -> Shift Arithmetic2/1, Shift Arithmetic/1, Gain1/1, Shift Arithmetic1/1

== system Sim_Forcing_003h_expe_infra5_full_control4/BEC (May 7, 2015)/CAN Send/If Action Subsystem1/Convert int to 4*uni8 3 ==
  in : Inport
  Gain{1..4} (4 alike) : Gain  ParameterDataType=fixdt(1, 16)  ParameterScaling=2^0  OutDataTypeMode=uint8  OutDataType=fixdt(1, 16)  OutScaling=2^0  OutDataTypeStr=uint8
  Mux : Mux
  Shift Arithmetic : simulink/Logic and Bit Operations/Shift Arithmetic  SystemSampleTime=-1  nBitShiftRight=8  nBinPtShiftRight=0
  Shift Arithmetic1 : simulink/Logic and Bit Operations/Shift Arithmetic  SystemSampleTime=-1  nBitShiftRight=16  nBinPtShiftRight=0
  Shift Arithmetic2 : simulink/Logic and Bit Operations/Shift Arithmetic  SystemSampleTime=-1  nBitShiftRight=24  nBinPtShiftRight=0
  out : Outport
  wires:
  in/1 -> Shift Arithmetic1/1, Gain1/1, Shift Arithmetic/1, Shift Arithmetic2/1
  Shift Arithmetic/1 -> Gain2/1
  Shift Arithmetic1/1 -> Gain3/1
  Shift Arithmetic2/1 -> Gain4/1
  Gain1/1 -> Mux/1
  Gain2/1 -> Mux/2
  Gain3/1 -> Mux/3
  Gain4/1 -> Mux/4
  Mux/1 -> out/1

== system Sim_Forcing_003h_expe_infra5_full_control4/BEC (May 7, 2015)/CAN Send/If Action Subsystem1/Convert int to 4*uni8 4 ==
  in : Inport
  Gain{1..4} (4 alike) : Gain  ParameterDataType=fixdt(1, 16)  ParameterScaling=2^0  OutDataTypeMode=uint8  OutDataType=fixdt(1, 16)  OutScaling=2^0  OutDataTypeStr=uint8
  Mux : Mux
  Shift Arithmetic : simulink/Logic and Bit Operations/Shift Arithmetic  SystemSampleTime=-1  nBitShiftRight=8  nBinPtShiftRight=0
  Shift Arithmetic1 : simulink/Logic and Bit Operations/Shift Arithmetic  SystemSampleTime=-1  nBitShiftRight=16  nBinPtShiftRight=0
  Shift Arithmetic2 : simulink/Logic and Bit Operations/Shift Arithmetic  SystemSampleTime=-1  nBitShiftRight=24  nBinPtShiftRight=0
  out : Outport
  wires:
  in/1 -> Shift Arithmetic1/1, Gain1/1, Shift Arithmetic/1, Shift Arithmetic2/1
  Shift Arithmetic/1 -> Gain2/1
  Shift Arithmetic1/1 -> Gain3/1
  Shift Arithmetic2/1 -> Gain4/1
  Gain1/1 -> Mux/1
  Gain2/1 -> Mux/2
  Gain3/1 -> Mux/3
  Gain4/1 -> Mux/4
  Mux/1 -> out/1

== system Sim_Forcing_003h_expe_infra5_full_control4/BEC (May 7, 2015)/CAN Send/If Action Subsystem1/Convert int to 4*uni8 5 ==
  in : Inport
  Gain{1..4} (4 alike) : Gain  ParameterDataType=fixdt(1, 16)  ParameterScaling=2^0  OutDataTypeMode=uint8  OutDataType=fixdt(1, 16)  OutScaling=2^0  OutDataTypeStr=uint8
  Mux : Mux
  Shift Arithmetic : simulink/Logic and Bit Operations/Shift Arithmetic  SystemSampleTime=-1  nBitShiftRight=8  nBinPtShiftRight=0
  Shift Arithmetic1 : simulink/Logic and Bit Operations/Shift Arithmetic  SystemSampleTime=-1  nBitShiftRight=16  nBinPtShiftRight=0
  Shift Arithmetic2 : simulink/Logic and Bit Operations/Shift Arithmetic  SystemSampleTime=-1  nBitShiftRight=24  nBinPtShiftRight=0
  out : Outport
  wires:
  Mux/1 -> out/1
  Gain4/1 -> Mux/4
  Gain3/1 -> Mux/3
  Gain2/1 -> Mux/2
  Gain1/1 -> Mux/1
  Shift Arithmetic2/1 -> Gain4/1
  Shift Arithmetic1/1 -> Gain3/1
  Shift Arithmetic/1 -> Gain2/1
  in/1 -> Shift Arithmetic2/1, Shift Arithmetic/1, Gain1/1, Shift Arithmetic1/1

== system Sim_Forcing_003h_expe_infra5_full_control4/BEC (May 7, 2015)/Software limit switches/Subsystem/If Action Subsystem ==
  dif : Inport  OutDataType=fixdt(1, 16)  OutScaling=2^0
  Inc : Inport  Port=2  OutDataType=fixdt(1, 16)  OutScaling=2^0
  Action Port : ActionPort  ActionType=then
  PSEA2 : Constant  Value=0  OutDataType=fixdt(1, 16)  OutScaling=2^0
  Switch : Switch  Criteria=u2 > Threshold  Threshold=1  OutDataType=fixdt(1, 16)  OutScaling=2^0
  Out1 : Outport  OutDataType=fixdt(1, 16)  OutScaling=2^0
  wires:
  PSEA2/1 -> Switch/3
  Switch/1 -> Out1/1
  Inc/1 -> Switch/1
  dif/1 -> Switch/2

== system Sim_Forcing_003h_expe_infra5_full_control4/BEC (May 7, 2015)/Software limit switches/Subsystem/If Action Subsystem1 ==
  Inc : Inport  OutDataType=fixdt(1, 16)  OutScaling=2^0
  dif : Inport  Port=2  OutDataType=fixdt(1, 16)  OutScaling=2^0
  Action Port : ActionPort  ActionType=else
  PSEA2 : Constant  Value=0  OutDataType=fixdt(1, 16)  OutScaling=2^0
  Switch : Switch  Threshold=1  OutDataType=fixdt(1, 16)  OutScaling=2^0
  Out1 : Outport  OutDataType=fixdt(1, 16)  OutScaling=2^0
  wires:
  dif/1 -> Switch/2
  Inc/1 -> Switch/1
  Switch/1 -> Out1/1
  PSEA2/1 -> Switch/3

== system Sim_Forcing_003h_expe_infra5_full_control4/BEC (May 7, 2015)/Software limit switches/Subsystem1/If Action Subsystem ==
  dif : Inport  OutDataType=fixdt(1, 16)  OutScaling=2^0
  Inc : Inport  Port=2  OutDataType=fixdt(1, 16)  OutScaling=2^0
  Action Port : ActionPort  ActionType=then
  PSEA2 : Constant  Value=0  OutDataType=fixdt(1, 16)  OutScaling=2^0
  Switch : Switch  Threshold=1  OutDataType=fixdt(1, 16)  OutScaling=2^0
  Out1 : Outport  OutDataType=fixdt(1, 16)  OutScaling=2^0
  wires:
  dif/1 -> Switch/2
  Inc/1 -> Switch/1
  Switch/1 -> Out1/1
  PSEA2/1 -> Switch/3

== system Sim_Forcing_003h_expe_infra5_full_control4/BEC (May 7, 2015)/Software limit switches/Subsystem1/If Action Subsystem1 ==
  Inc : Inport  OutDataType=fixdt(1, 16)  OutScaling=2^0
  dif : Inport  Port=2  OutDataType=fixdt(1, 16)  OutScaling=2^0
  Action Port : ActionPort  ActionType=else
  PSEA2 : Constant  Value=0  OutDataType=fixdt(1, 16)  OutScaling=2^0
  Switch : Switch  Threshold=1  OutDataType=fixdt(1, 16)  OutScaling=2^0
  Out1 : Outport  OutDataType=fixdt(1, 16)  OutScaling=2^0
  wires:
  PSEA2/1 -> Switch/3
  Switch/1 -> Out1/1
  Inc/1 -> Switch/1
  dif/1 -> Switch/2

== system Sim_Forcing_003h_expe_infra5_full_control4/BEC (May 7, 2015)/Software limit switches/Subsystem2/If Action Subsystem ==
  dif : Inport  OutDataType=fixdt(1, 16)  OutScaling=2^0
  Inc : Inport  Port=2  OutDataType=fixdt(1, 16)  OutScaling=2^0
  Action Port : ActionPort  ActionType=then
  PSEA2 : Constant  Value=0  OutDataType=fixdt(1, 16)  OutScaling=2^0
  Switch : Switch  Threshold=1  OutDataType=fixdt(1, 16)  OutScaling=2^0
  Out1 : Outport  OutDataType=fixdt(1, 16)  OutScaling=2^0
  wires:
  PSEA2/1 -> Switch/3
  Switch/1 -> Out1/1
  Inc/1 -> Switch/1
  dif/1 -> Switch/2

== system Sim_Forcing_003h_expe_infra5_full_control4/BEC (May 7, 2015)/Software limit switches/Subsystem2/If Action Subsystem1 ==
  Inc : Inport  OutDataType=fixdt(1, 16)  OutScaling=2^0
  dif : Inport  Port=2  OutDataType=fixdt(1, 16)  OutScaling=2^0
  Action Port : ActionPort  ActionType=else
  PSEA2 : Constant  Value=0  OutDataType=fixdt(1, 16)  OutScaling=2^0
  Switch : Switch  Threshold=1  OutDataType=fixdt(1, 16)  OutScaling=2^0
  Out1 : Outport  OutDataType=fixdt(1, 16)  OutScaling=2^0
  wires:
  dif/1 -> Switch/2
  Inc/1 -> Switch/1
  Switch/1 -> Out1/1
  PSEA2/1 -> Switch/3

== system Sim_Forcing_003h_expe_infra5_full_control4/BEC (May 7, 2015)/Software limit switches/Subsystem3/If Action Subsystem ==
  dif : Inport  OutDataType=fixdt(1, 16)  OutScaling=2^0
  Inc : Inport  Port=2  OutDataType=fixdt(1, 16)  OutScaling=2^0
  Action Port : ActionPort  ActionType=then
  PSEA2 : Constant  Value=0  OutDataType=fixdt(1, 16)  OutScaling=2^0
  Switch : Switch  Threshold=1  OutDataType=fixdt(1, 16)  OutScaling=2^0
  Out1 : Outport  OutDataType=fixdt(1, 16)  OutScaling=2^0
  wires:
  dif/1 -> Switch/2
  Inc/1 -> Switch/1
  Switch/1 -> Out1/1
  PSEA2/1 -> Switch/3
